simulink library "Window_Ventilation"  (R2018b)
settings: Solver=ode45  StartTime=0.0  StopTime=10.0  RelTol=1e-3  EnableMultiTasking=on
settings Model: Creator=lena.frank  LastModifiedBy=drhf
settings DataIOCC: LimitDataPoints=on  SaveFormat=Array  SignalLoggingSaveFormat=ModelDataLogs
settings OptimizationCC: ExpressionDepthLimit=2147483647  LifeSpan=inf
settings DebuggingCC: UnderspecifiedInitializationDetection=Classic  MergeDetectMultiDrivingBlocksExec=none  SolverPrmCheckMsg=warning  FcnCallInpInsideContextMsg=warning  StateNameClashWarn=warning  SFUnexpectedBacktrackingDiag=warning  SFNoUnconditionalDefaultTransitionDiag=warning  SFExecutionAtInitializationDiag=none
settings HardwareCC: ProdBitPerPointer=32  ProdBitPerSizeT=32  ProdBitPerPtrDiffT=32  ProdLargestAtomicFloat=None  ProdIntDivRoundTo=Undefined  ProdEndianess=Unspecified  ProdWordSize=32  ProdHWDeviceType=32-bit Generic
settings ModelReferenceCC: PropagateSignalLabelsOutOfModel=off
settings SFSimCC: SimUseLocalCustomCode=off
settings RTWCC: RTWUseLocalCustomCode=off
settings CodeAppCC: StateflowObjectComments=on
settings GRTTargetCC: TargetLangStandard=C89/C90 (ANSI)  GeneratePreprocessorConditionals=Disable all  CombineOutputUpdateFcns=off  GRTInterface=on
settings ConfigComp: CovMetricSettings=dw  CovHtmlReporting=on  CovSaveCumulativeToWorkspaceVar=on  CovSaveSingleToWorkspaceVar=on  CovExternalEMLEnable=off

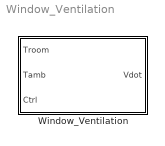
== system Window_Ventilation ==
  Window_Ventilation : Subsystem  mask(window ventilation){alpha=10, H=1.2, W=1, Nwin=4}
      mask prompts: alpha "maximal opening angle (°)"; H "height of window (m)"; W "width of window (m)"; Nwin "Number of windows"
      mask help: Simulates the free driven ventilation through a window with an opening angle of [0,1]* max. angle. Valid for angles between 8° and 180°. Output is the VOLUME FLOW RATE in m^3/s. Calculation based on Weber.
      mask Help: web(fullfile(path_carnot('help'),'Window_Ventilation.html'),'-helpbrowser')
      mask TypeOptions Nwin: NumberOfWindows/Gain
      mask Display:
      | plot(0,10,90,80,[20 70 70 20 20],[20 20 70 70 20],...
      |     [20 70 80 30 20],[20 20 65 65 20])

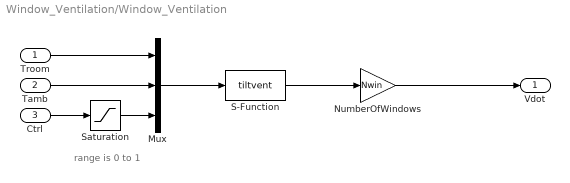
== system Window_Ventilation/Window_Ventilation ==
  note: range is 0 to 1
  Troom : Inport
  Tamb : Inport  Port=2
  Ctrl : Inport  Port=3
  Mux : Mux  Inputs=3
  NumberOfWindows : Gain  Gain=Nwin
  S-Function : S-Function  FunctionName=tiltvent  Parameters=alpha, H, W  SFunctionDeploymentMode=off  EnableBusSupport=off
  Saturation : Saturate  UpperLimit=1  LowerLimit=0
  Vdot : Outport
  wires:
  NumberOfWindows/1 -> Vdot/1
  Tamb/1 -> Mux/2
  Ctrl/1 -> Saturation/1
  S-Function/1 -> NumberOfWindows/1
  Mux/1 -> S-Function/1
  Troom/1 -> Mux/1
  Saturation/1 -> Mux/3
